simulink model "psbnetsim1"  (Simulink 6.0)
settings: Solver=ode15s  SolverMode=SingleTasking  StartTime=0.0  StopTime=0.1  RelTol=1e-3  AbsTol=0.01
libraries: powerlib2 x10
settings Model: Creator=patrice  LastModifiedBy=batserve  ExtModeTrigMode=oneshot  ExtModeArmWhenConnect=off  ExtModeAutoUpdateStatusClock=off
settings SolverCC: MaxOrder=2
settings DataIOCC: LimitDataPoints=off  SignalLoggingName=sigsOut
settings OptimizationCC: BooleanDataType=off
settings DebuggingCC: SolverPrmCheckMsg=none
settings HardwareCC: TargetUnknown=on
settings RTWCC: TemplateMakefile=grt_unix.tmf

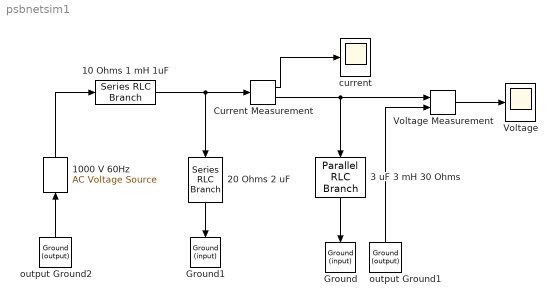
== system psbnetsim1 ==
  10 Ohms 1 mH 1uF : powerlib2/Elements/Series RLC Branch  Tag=PoWeRsYsTeMbLoCk  a=10  b=1e-03  c=1e-06  mesure=None  PSBOutputType=1
  1000 V 60Hz : powerlib2/Electrical Sources/AC Voltage Source  Tag=PoWeRsYsTeMbLoCk  Description=source block  Orientation=up  A=1000  P=0  F=60  stime=0  mesure=None  PSBOutputType=1
  20 Ohms 2 uF : powerlib2/Elements/Series RLC Branch  Tag=PoWeRsYsTeMbLoCk  Orientation=down  a=20  b=0  c=2e-06  mesure=None  PSBOutputType=1
  3 uF 3 mH 30 Ohms : powerlib2/Elements/Parallel RLC Branch  Tag=PoWeRsYsTeMbLoCk  Orientation=down  a=30  b=3e-03  c=3e-06  mesure=None  PSBOutputType=1
  Current Measurement : powerlib2/Measurements/Current Measurement  Tag=PoWeRsYsTeMmEaSuReMeNt  PhasorSimulation=off  OutputType=Magnitude  PSBOutputType=01  PSBequivalent=0
  Ground : powerlib2/Connectors/Ground (input)  Tag=PoWeRsYsTeMbLoCk  Orientation=down
  Ground1 : powerlib2/Connectors/Ground (input)  Tag=PoWeRsYsTeMbLoCk  Orientation=down
  Voltage : Scope
      settings: TickLabels=on  YMin=-0.5  YMax=0.5  DataFormat=Array  MaxDataPoints=100000
  Voltage Measurement : powerlib2/Measurements/Voltage Measurement  Tag=PoWeRsYsTeMmEaSuReMeNt  PhasorSimulation=off  OutputType=Magnitude  PSBOutputType=0  PSBequivalent=0
  current : Scope
      settings: TickLabels=on  YMin=-0.5  YMax=0.5  DataFormat=Array  MaxDataPoints=100000
  output Ground1 : powerlib2/Connectors/Ground (output)  Tag=PoWeRsYsTeMbLoCk  Orientation=up  PSBOutputType=1
  output Ground2 : powerlib2/Connectors/Ground (output)  Tag=PoWeRsYsTeMbLoCk  Orientation=up  PSBOutputType=1
  wires:
  output Ground2/1 -> 1000 V 60Hz/1
  1000 V 60Hz/1 -> 10 Ohms 1 mH 1uF/1
  20 Ohms 2 uF/1 -> Ground1/1
  3 uF 3 mH 30 Ohms/1 -> Ground/1
  10 Ohms 1 mH 1uF/1 -> 20 Ohms 2 uF/1, Current Measurement/1
  Current Measurement/2 -> 3 uF 3 mH 30 Ohms/1, Voltage Measurement/1
  output Ground1/1 -> Voltage Measurement/2
  Current Measurement/1 -> current/1
  Voltage Measurement/1 -> Voltage/1
